simulink model "FullSystemSim"  (R2017b)
settings: Solver=ode45  StartTime=t0  StopTime=tf  RelTol=1e-6  AbsTol=1e-6
values from neighbouring files (symbols this model uses):
  I_MAG1 = 1    [runAll.m]
  I_MAG2 = 1    [runAll.m]
  I_MAG3 = 1    [runAll.m]
  I_MAG4 = 1    [runAll.m]
  iBeamThick = 0.313*(0.0254)    (= 0.0079502)    [runAll.m]
  Tx = 0    [runAll.m]
  Tx_err = 0    [runAll.m]
  Ty = 0    [runAll.m]
  Ty_err = 0    [runAll.m]
  Tz = 0    [runAll.m]
  Tz_err = 0    [runAll.m]
libraries: HyperloopSimLibrary x1, sharedtransform x1
settings Model: Creator=hh  LastModifiedBy=hh

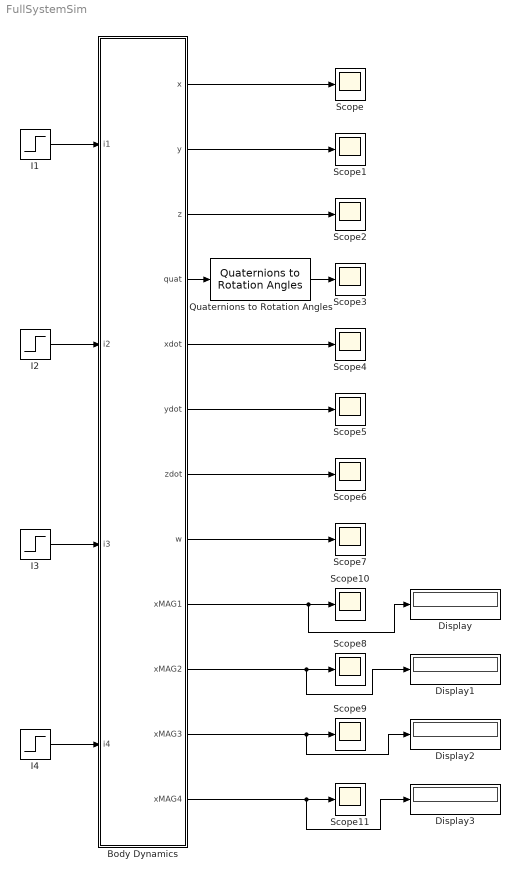
== system FullSystemSim ==
  Body Dynamics : Subsystem
  Display{,1..3} (4 alike) : Display
  I1 : Step  Time=0  After=I_MAG1  SampleTime=0
  I2 : Step  Time=0  After=I_MAG2  SampleTime=0
  I3 : Step  Time=0  After=I_MAG3  SampleTime=0
  I4 : Step  Time=0  After=I_MAG4  SampleTime=0
  Quaternions to Rotation Angles : sharedtransform/Quaternions to Rotation Angles  rotationOrder=ZYX
      settings: SourceProductBaseCode=AE
  Scope{,1..11} (12 alike) : Scope
  wires:
  Quaternions to Rotation Angles/1 -> Scope3/1
  Body Dynamics/11(xMAG3) -> Display2/1, Scope9/1
  Body Dynamics/12(xMAG4) -> Scope11/1, Display3/1
  Body Dynamics/10(xMAG2) -> Scope8/1, Display1/1
  Body Dynamics/9(xMAG1) -> Scope10/1, Display/1
  I1/1 -> Body Dynamics/1(i1)
  I2/1 -> Body Dynamics/2(i2)
  I3/1 -> Body Dynamics/3(i3)
  I4/1 -> Body Dynamics/4(i4)
  Body Dynamics/1(x) -> Scope/1
  Body Dynamics/2(y) -> Scope1/1
  Body Dynamics/3(z) -> Scope2/1
  Body Dynamics/4(quat) -> Quaternions to Rotation Angles/1
  Body Dynamics/5(xdot) -> Scope4/1
  Body Dynamics/6(ydot) -> Scope5/1
  Body Dynamics/7(zdot) -> Scope6/1
  Body Dynamics/8(w) -> Scope7/1

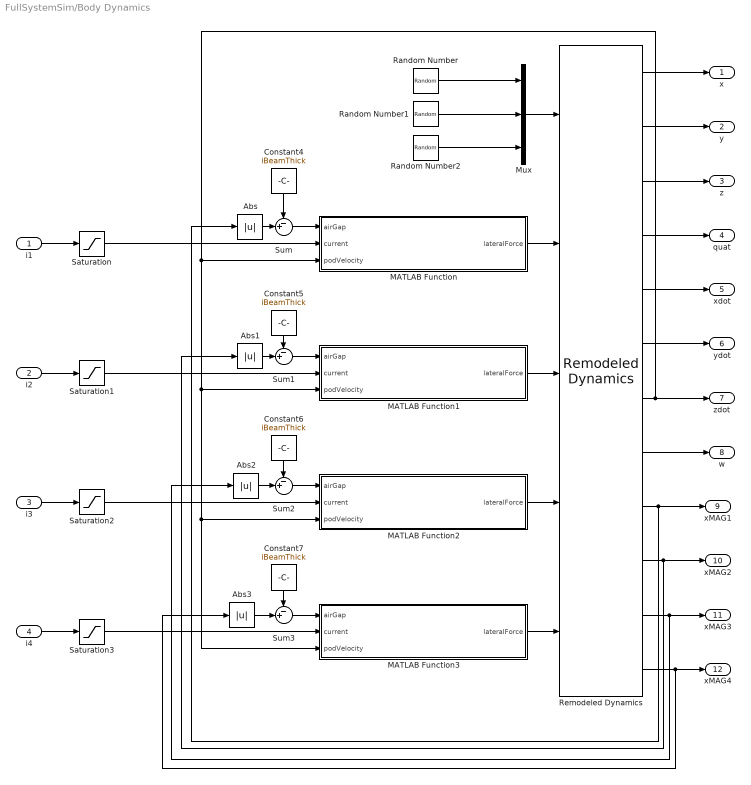
== system FullSystemSim/Body Dynamics ==
  i1 : Inport
  i2 : Inport  Port=2
  i3 : Inport  Port=3
  i4 : Inport  Port=4
  Abs{,1..3} (4 alike) : Abs
  Constant{4..7} (4 alike) : Constant  Value=iBeamThick
  MATLAB Function : MATLAB Function  TreatAsAtomicUnit=on
  MATLAB Function1 : MATLAB Function  TreatAsAtomicUnit=on
  MATLAB Function2 : MATLAB Function  TreatAsAtomicUnit=on
  MATLAB Function3 : MATLAB Function  TreatAsAtomicUnit=on
  Mux : Mux  Inputs=3
  Random Number : RandomNumber  Mean=Tx  Variance=Tx_err^2  SampleTime=0.1
  Random Number1 : RandomNumber  Mean=Ty  Variance=Ty_err^2  SampleTime=0.1
  Random Number2 : RandomNumber  Mean=Tz  Variance=Tz_err^2  SampleTime=0.1
  Remodeled Dynamics : HyperloopSimLibrary/Remodeled Dynamics
      link override Solid: ExtGeomFileName=D:\Google Drive\Cornell Engineering\Course Work\Projects\Cornell Hyperloop\Hyperloop Control Simulation\HyperloopCAD_2018\Master Assembly\pod.stp
  Saturation{,1..3} (4 alike) : Saturate  UpperLimit=1  LowerLimit=-1
  Sum{,1..3} (4 alike) : Sum  Inputs=-+|
  x : Outport
  y : Outport  Port=2
  z : Outport  Port=3
  quat : Outport  Port=4
  xdot : Outport  Port=5
  ydot : Outport  Port=6
  zdot : Outport  Port=7
  w : Outport  Port=8
  xMAG1 : Outport  Port=9
  xMAG2 : Outport  Port=10
  xMAG3 : Outport  Port=11
  xMAG4 : Outport  Port=12
  wires:
  Abs/1 -> Sum/2
  MATLAB Function2/1(lateralForce) -> Remodeled Dynamics/4
  i2/1 -> Saturation1/1
  i1/1 -> Saturation/1
  Remodeled Dynamics/1 -> x/1
  Remodeled Dynamics/2 -> y/1
  Mux/1 -> Remodeled Dynamics/1
  Remodeled Dynamics/3 -> z/1
  Remodeled Dynamics/6 -> ydot/1
  Random Number/1 -> Mux/1
  Remodeled Dynamics/7 -> zdot/1, MATLAB Function3/3(podVelocity), MATLAB Function2/3(podVelocity), MATLAB Function1/3(podVelocity), MATLAB Function/3(podVelocity)
  MATLAB Function/1(lateralForce) -> Remodeled Dynamics/2
  i3/1 -> Saturation2/1
  Random Number1/1 -> Mux/2
  i4/1 -> Saturation3/1
  Remodeled Dynamics/9 -> xMAG1/1, Abs/1
  Remodeled Dynamics/8 -> w/1
  Remodeled Dynamics/4 -> quat/1
  Remodeled Dynamics/5 -> xdot/1
  Random Number2/1 -> Mux/3
  Abs1/1 -> Sum1/2
  Abs3/1 -> Sum3/2
  Abs2/1 -> Sum2/2
  Remodeled Dynamics/11 -> xMAG3/1, Abs2/1
  Constant6/1 -> Sum2/1
  Sum2/1 -> MATLAB Function2/1(airGap)
  Sum/1 -> MATLAB Function/1(airGap)
  Constant7/1 -> Sum3/1
  Sum3/1 -> MATLAB Function3/1(airGap)
  Constant4/1 -> Sum/1
  MATLAB Function1/1(lateralForce) -> Remodeled Dynamics/3
  Remodeled Dynamics/12 -> xMAG4/1, Abs3/1
  MATLAB Function3/1(lateralForce) -> Remodeled Dynamics/5
  Constant5/1 -> Sum1/1
  Sum1/1 -> MATLAB Function1/1(airGap)
  Remodeled Dynamics/10 -> xMAG2/1, Abs1/1
  Saturation/1 -> MATLAB Function/2(current)
  Saturation1/1 -> MATLAB Function1/2(current)
  Saturation2/1 -> MATLAB Function2/2(current)
  Saturation3/1 -> MATLAB Function3/2(current)

== matlab function FullSystemSim/Body Dynamics/MATLAB Function1 ==
  data: airGap input; lateralForce output; current input; podVelocity input
function lateralForce  = computeLateralForce(airGap,current,podVelocity)

%i-beam constants
alumResistivity = 100 * (3.99e-006); %ohm-m
alumConducitivity = 1/alumResistivity; %S/m
iBeamThick = 0.313*(0.0254); %meters
%relative permeability
mu = 4*pi*10^(-7)*200000;

% podVelocity = 200*(0.44704); %meters per second

%constants chosen for simulation purposes
windings = 1000;
crossSectArea = 4.5e-3;

%compute lateral force for one magnet using magnetLateralForce Module
[lateralForce] = magnetLateralForce(alumConducitivity, ...
mu, iBeamThick, podVelocity, airGap, windings, current, crossSectArea);
end

function [lateralForce] = magnetLateralForce(metalConductivity, mu, beamThick, ...
podVelocity, airGap, windings, current, crossSectArea)
%Parameters:
%conductivity of i-beam
%relative permeability of i-beam
%thickness of i-beam
%pod velocity 
%distance between magnet and i-beam
%number of solenoid windings 
%current supplied to the solenoid
%cross sectional area of the solenoid

%Vacuum Permeability
mu0 = 4*pi*10^(-7);

%Contributions to p from solenoid and the core
psolenoid = windings*current*crossSectArea;
pcore = windings*current*crossSectArea*(1-(mu0/mu));
p=psolenoid + pcore;

%mirror image velocity (w). material property
w = 2/(beamThick*mu*mu0*metalConductivity);

%relationship between close magnet and far magnet force
lateralForce= ((3*mu0*p^2)./(32*pi*airGap.^4) ) * (1- w/sqrt(podVelocity^2 + w^2));
end

== matlab function FullSystemSim/Body Dynamics/MATLAB Function ==
  data: airGap input; lateralForce output; current input; podVelocity input
function lateralForce  = computeLateralForce(airGap,current,podVelocity)

%i-beam constants
alumResistivity = 100 * (3.99e-006); %ohm-m
alumConducitivity = 1/alumResistivity; %S/m
iBeamThick = 0.313*(0.0254); %meters
%relative permeability
mu = 4*pi*10^(-7)*200000;

% podVelocity = 200*(0.44704); %meters per second

%constants chosen for simulation purposes
windings = 1000;
crossSectArea = 4.5e-3;

%compute lateral force for one magnet using magnetLateralForce Module
[lateralForce] = magnetLateralForce(alumConducitivity, ...
mu, iBeamThick, podVelocity, airGap, windings, current, crossSectArea);
end

function [lateralForce] = magnetLateralForce(metalConductivity, mu, beamThick, ...
podVelocity, airGap, windings, current, crossSectArea)
%Parameters:
%conductivity of i-beam
%relative permeability of i-beam
%thickness of i-beam
%pod velocity 
%distance between magnet and i-beam
%number of solenoid windings 
%current supplied to the solenoid
%cross sectional area of the solenoid

%Vacuum Permeability
mu0 = 4*pi*10^(-7);

%Contributions to p from solenoid and the core
psolenoid = windings*current*crossSectArea;
pcore = windings*current*crossSectArea*(1-(mu0/mu));
p=psolenoid + pcore;

%mirror image velocity (w). material property
w = 2/(beamThick*mu*mu0*metalConductivity);

%relationship between close magnet and far magnet force
lateralForce= ((3*mu0*p^2)./(32*pi*airGap.^4) ) * (1- w/sqrt(podVelocity.^2 + w^2));
end

== matlab function FullSystemSim/Body Dynamics/MATLAB Function2 ==
  data: airGap input; lateralForce output; current input; podVelocity input
function lateralForce  = computeLateralForce(airGap,current,podVelocity)

%i-beam constants
alumResistivity = 100 * (3.99e-006); %ohm-m
alumConducitivity = 1/alumResistivity; %S/m
iBeamThick = 0.313*(0.0254); %meters
%relative permeability
mu = 4*pi*10^(-7)*200000;

% podVelocity = 200*(0.44704); %meters per second

%constants chosen for simulation purposes
windings = 1000;
crossSectArea = 4.5e-3;

%compute lateral force for one magnet using magnetLateralForce Module
[lateralForce] = magnetLateralForce(alumConducitivity, ...
mu, iBeamThick, podVelocity, airGap, windings, current, crossSectArea);
end

function [lateralForce] = magnetLateralForce(metalConductivity, mu, beamThick, ...
podVelocity, airGap, windings, current, crossSectArea)
%Parameters:
%conductivity of i-beam
%relative permeability of i-beam
%thickness of i-beam
%pod velocity 
%distance between magnet and i-beam
%number of solenoid windings 
%current supplied to the solenoid
%cross sectional area of the solenoid

%Vacuum Permeability
mu0 = 4*pi*10^(-7);

%Contributions to p from solenoid and the core
psolenoid = windings*current*crossSectArea;
pcore = windings*current*crossSectArea*(1-(mu0/mu));
p=psolenoid + pcore;

%mirror image velocity (w). material property
w = 2/(beamThick*mu*mu0*metalConductivity);

%relationship between close magnet and far magnet force
lateralForce= ((3*mu0*p^2)./(32*pi*airGap.^4) ) * (1- w/sqrt(podVelocity^2 + w^2));
end

== matlab function FullSystemSim/Body Dynamics/MATLAB Function3 ==
  data: airGap input; lateralForce output; current input; podVelocity input
function lateralForce  = computeLateralForce(airGap,current,podVelocity)

%i-beam constants
alumResistivity = 100 * (3.99e-006); %ohm-m
alumConducitivity = 1/alumResistivity; %S/m
iBeamThick = 0.313*(0.0254); %meters
%relative permeability
mu = 4*pi*10^(-7)*200000;

% podVelocity = 200*(0.44704); %meters per second

%constants chosen for simulation purposes
windings = 1000;
crossSectArea = 4.5e-3;

%compute lateral force for one magnet using magnetLateralForce Module
[lateralForce] = magnetLateralForce(alumConducitivity, ...
mu, iBeamThick, podVelocity, airGap, windings, current, crossSectArea);
end

function [lateralForce] = magnetLateralForce(metalConductivity, mu, beamThick, ...
podVelocity, airGap, windings, current, crossSectArea)
%Parameters:
%conductivity of i-beam
%relative permeability of i-beam
%thickness of i-beam
%pod velocity 
%distance between magnet and i-beam
%number of solenoid windings 
%current supplied to the solenoid
%cross sectional area of the solenoid

%Vacuum Permeability
mu0 = 4*pi*10^(-7);

%Contributions to p from solenoid and the core
psolenoid = windings*current*crossSectArea;
pcore = windings*current*crossSectArea*(1-(mu0/mu));
p=psolenoid + pcore;

%mirror image velocity (w). material property
w = 2/(beamThick*mu*mu0*metalConductivity);

%relationship between close magnet and far magnet force
lateralForce= ((3*mu0*p^2)./(32*pi*airGap.^4) ) * (1- w/sqrt(podVelocity^2 + w^2));
end
